simulink model "test"  (R2023b)
settings: Solver=VariableStepAuto  StartTime=0.0  StopTime=10.0  RelTol=1e-3
model workspace (MAT data in the model file):
  k = Simulink.Parameter
  k.Value = 2
  k.DataType = 'auto'
  k.Complexity = 'real'
  k.Dimensions = [1 1]
  x = Simulink.Signal
  x.DataType = 'auto'
  x.Dimensions = -1
  x.DimensionsMode = 'auto'
  x.Complexity = 'auto'
  x.SampleTime = -1
  x.SamplingMode = 'auto'
  y = Simulink.Signal
  y.DataType = 'auto'
  y.Dimensions = -1
  y.DimensionsMode = 'auto'
  y.Complexity = 'auto'
  y.SampleTime = -1
  y.SamplingMode = 'auto'
  z = Simulink.Signal
  z.DataType = 'auto'
  z.Dimensions = -1
  z.DimensionsMode = 'auto'
  z.Complexity = 'auto'
  z.SampleTime = -1
  z.SamplingMode = 'auto'
settings Model: Creator=zhaop  LastModifiedBy=zhaop

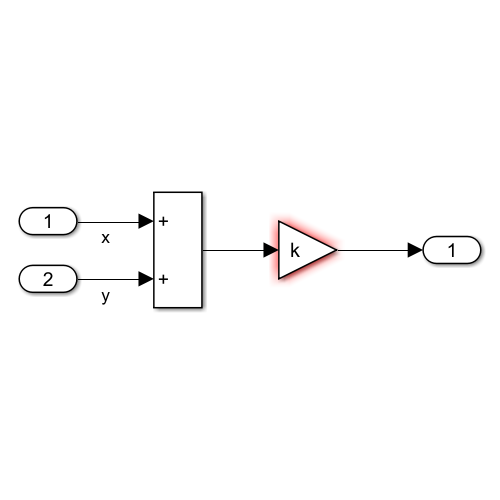
[thumbnail: Simulink's stored preview of the top-level diagram]
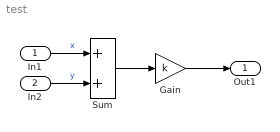
== system test ==
  In1 : Inport
  In2 : Inport  Port=2
  Gain : Gain  Gain=k
  Sum : Sum
  Out1 : Outport
  wires:
  In1/1 -> Sum/1  "x"
  Sum/1 -> Gain/1
  Gain/1 -> Out1/1
  In2/1 -> Sum/2  "y"
